simulink model "SelectiveHarmonicsEliminationfor1phbridgeinverter"  (R2023a)
settings: Solver=VariableStepAuto  StartTime=0.0  StopTime=0.2  RelTol=1e-3
values from neighbouring files (symbols this model uses):
  alpha = [alpha1;alpha2;alpha3;alpha4;alpha5]*180/pi    [SHEnewtonraphson.m]
libraries: spsIGBTDiodeLib x4, simulink x2, spsDCVoltageSourceLib x1, spsGroundLib x1, spsSeriesRLCBranchLib x1, spsVoltageMeasurementLib x1, sps_lib x1
settings Model: Creator=User  LastModifiedBy=User

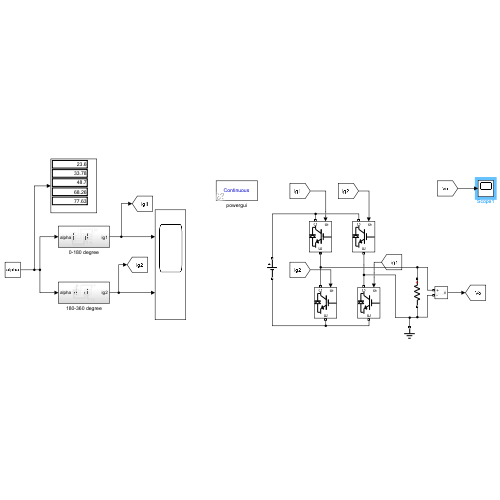
[thumbnail: Simulink's stored preview of the top-level diagram]
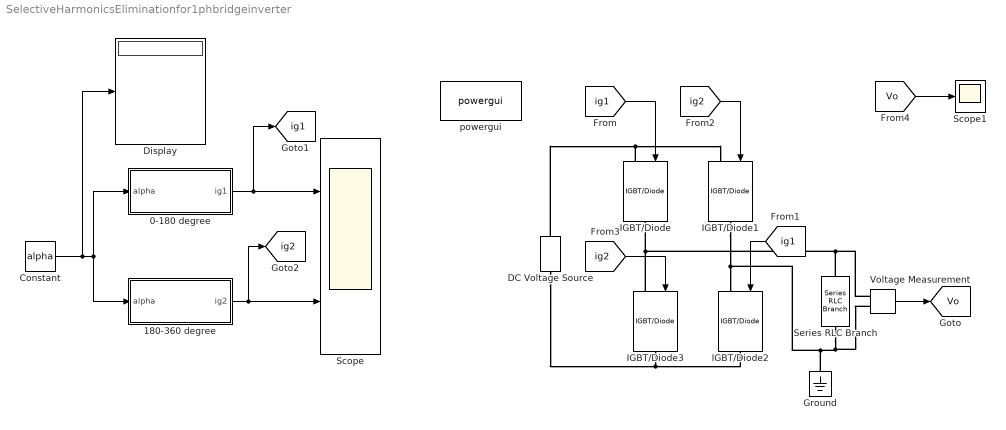
== system SelectiveHarmonicsEliminationfor1phbridgeinverter ==
  0-180 degree : Subsystem
  180-360 degree : Subsystem
  Constant : Constant  Value=alpha
  DC Voltage Source : spsDCVoltageSourceLib/DC Voltage Source  Amplitude=200  Measurements=None
  Display : Display
  Ground : spsGroundLib/Ground  LConnTagsString=a
  IGBT/Diode{,1..3} (4 alike) : spsIGBTDiodeLib/IGBT//Diode  Ron=1e-3  Rs=1e5  Cs=inf  Measurements=off
  Scope : Scope  NumInputPorts=2
  Scope1 : Scope
  Series RLC Branch : spsSeriesRLCBranchLib/Series RLC Branch  LConnTagsString=__new0  RConnTagsString=__new0  BranchType=R  Resistance=10  Inductance=1e-3  SetiL0=off  InitialCurrent=0  Capacitance=1e-6  Setx0=off  InitialVoltage=0  Measurements=None
  Voltage Measurement : spsVoltageMeasurementLib/Voltage Measurement  PhasorSimulation=off  OutputType=Complex  PSBequivalent=0
  powergui : sps_lib/powergui  Priority=1  SimulationMode=Continuous  SampleTime=50e-6  frequency=60  Iterations=50  frequencyindice=0  Pbase=100e6  ErrMax=1e-4  UnitsV=kV  UnitsW=MW  buscounter=0  FunctionMessages=off  echomessages=off  EnableUseOfTLC=off  CurrentSourceSwitches=off  DisableSnubberDevices=off  DisableRonSwitches=off  DisableVfSwitches=off  DisplayEquations=off  AutomaticDiscreteSolvers=off  SolverType=Tustin/Backward Euler (TBE)  Interpol=off  ExternalGateDelay=off  methode=off  Ts=100  x0status=blocks  SPID=on  SwTol=0  HookPort=off  NonlinearTolerance=1e-4  nMaxIteration=100  ContinueOnMaxIteration=off  RestoreLinks=warning  ResistiveCurrentMeasurement=off  Frange=[0:2:500]  Ylog=off  Xlog=on  ShowGrid=off  save=off  variable=ZData  structure=0  ZoomFFT=off  StartTime=0.0  cycles=1  DisplayStyle=1  fundamental=60  FreqAxis=off  MaxFrequency=1000  frequencyindicesteady=1  RmsSteady=1  display=off
  tag scope: Vo=global, ig1=global, ig2=global
  wires:
  Voltage Measurement/1 -> [Vo]
  Constant/1 -> Display/1, 180-360 degree/1(alpha), 0-180 degree/1(alpha)
  180-360 degree/1(ig2) -> Scope/2, [ig2]
  0-180 degree/1(ig1) -> [ig1], Scope/1
  [ig1] -> IGBT/Diode/1
  [ig1] -> IGBT/Diode2/1
  [ig2] -> IGBT/Diode1/1
  [ig2] -> IGBT/Diode3/1
  [Vo] -> Scope1/1
  connections:
  IGBT/Diode1/RConn1 -- Ground/LConn1 -- Voltage Measurement/LConn2 -- Series RLC Branch/RConn1 -- IGBT/Diode2/LConn1
  IGBT/Diode3/LConn1 -- Series RLC Branch/LConn1 -- Voltage Measurement/LConn1 -- IGBT/Diode/RConn1
  IGBT/Diode/LConn1 -- IGBT/Diode1/LConn1 -- DC Voltage Source/RConn1
  IGBT/Diode3/RConn1 -- IGBT/Diode2/RConn1 -- DC Voltage Source/LConn1

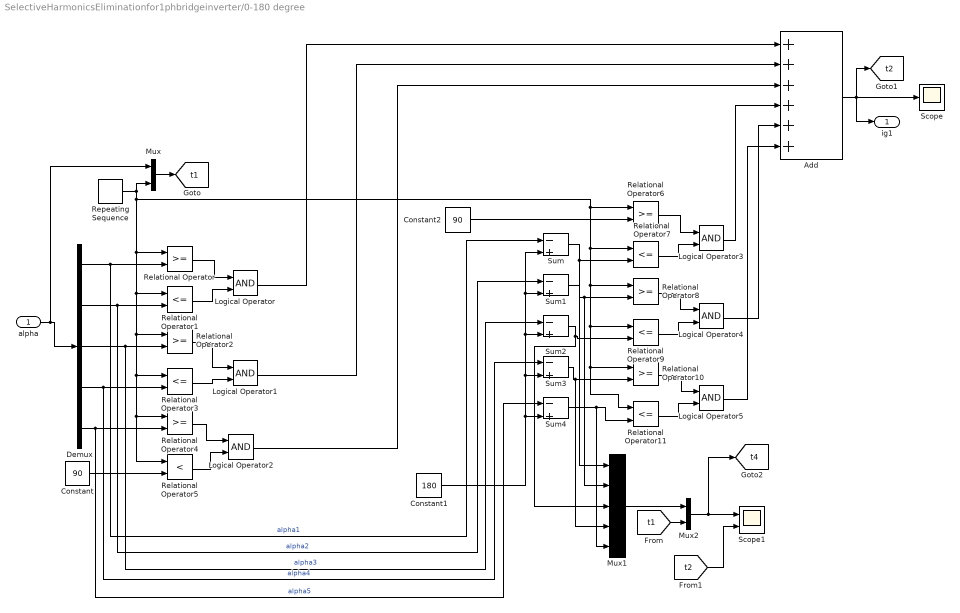
== system SelectiveHarmonicsEliminationfor1phbridgeinverter/0-180 degree ==
  alpha : Inport
  Add : Sum  Inputs=++++++  OutDataTypeStr=Inherit: Inherit via back propagation
  Constant : Constant  Value=90
  Constant1 : Constant  Value=180
  Constant2 : Constant  Value=90
  Demux : Demux  Outputs=5
  Logical Operator{,1..5} (6 alike) : Logic  AllPortsSameDT=off  OutDataTypeStr=boolean
  Mux : Mux  Inputs=2
  Mux1 : Mux  Inputs=5
  Mux2 : Mux  Inputs=2
  Relational Operator{,2,4,6,8,10} (6 alike) : RelationalOperator  OutDataTypeStr=boolean  RndMeth=Simplest  InputSameDT=off
  Relational Operator{1,3,7,9,11} (5 alike) : RelationalOperator  Operator=<=  OutDataTypeStr=boolean  RndMeth=Simplest  InputSameDT=off
  Relational Operator5 : RelationalOperator  Operator=<  OutDataTypeStr=boolean  RndMeth=Simplest  InputSameDT=off
  Repeating Sequence : simulink/Sources/Repeating Sequence  rep_seq_t=[0 1]*0.02  rep_seq_y=[0 360]
  Scope : Scope
  Scope1 : Scope  NumInputPorts=2
  Sum{,1..4} (5 alike) : Sum  Inputs=|-+
  ig1 : Outport
  tag scope: t1=global, t2=global, t4=global
  wires:
  alpha/1 -> Mux/1, Demux/1
  Relational Operator/1 -> Logical Operator/1
  Relational Operator1/1 -> Logical Operator/2
  Relational Operator2/1 -> Logical Operator1/1
  Relational Operator3/1 -> Logical Operator1/2
  Relational Operator4/1 -> Logical Operator2/1
  Relational Operator5/1 -> Logical Operator2/2
  Demux/1 -> Relational Operator/2, Sum/1  "alpha1"
  Demux/2 -> Sum1/1, Relational Operator1/2  "alpha2"
  Demux/3 -> Sum2/1, Relational Operator2/2  "alpha3"
  Demux/4 -> Sum3/1, Relational Operator3/2  "alpha4"
  Demux/5 -> Sum4/1, Relational Operator4/2  "alpha5"
  Constant/1 -> Relational Operator5/2
  Mux/1 -> [t1]
  Repeating Sequence/1 -> Mux/2, Relational Operator5/1, Relational Operator4/1, Relational Operator3/1, Relational Operator2/1, Relational Operator1/1, Relational Operator/1, Relational Operator10/1, Relational Operator11/1, Relational Operator9/1, Relational Operator8/1, Relational Operator7/1, Relational Operator6/1
  Constant1/1 -> Sum/2, Sum1/2, Sum2/2, Sum3/2, Sum4/2
  Relational Operator6/1 -> Logical Operator3/1
  Relational Operator7/1 -> Logical Operator3/2
  Relational Operator8/1 -> Logical Operator4/1
  Relational Operator9/1 -> Logical Operator4/2
  Relational Operator10/1 -> Logical Operator5/1
  Relational Operator11/1 -> Logical Operator5/2
  Sum/1 -> Mux1/1, Relational Operator7/2
  Constant2/1 -> Relational Operator6/2
  Sum1/1 -> Mux1/2, Relational Operator8/2
  Sum2/1 -> Mux1/3, Relational Operator9/2
  Sum3/1 -> Mux1/4, Relational Operator10/2
  Sum4/1 -> Mux1/5, Relational Operator11/2
  Logical Operator/1 -> Add/1
  Logical Operator1/1 -> Add/2
  Logical Operator2/1 -> Add/3
  Logical Operator3/1 -> Add/4
  Logical Operator4/1 -> Add/5
  Logical Operator5/1 -> Add/6
  Add/1 -> ig1/1, Scope/1, [t2]
  Mux1/1 -> Mux2/1
  [t1] -> Mux2/2
  Mux2/1 -> [t4], Scope1/1
  [t2] -> Scope1/2

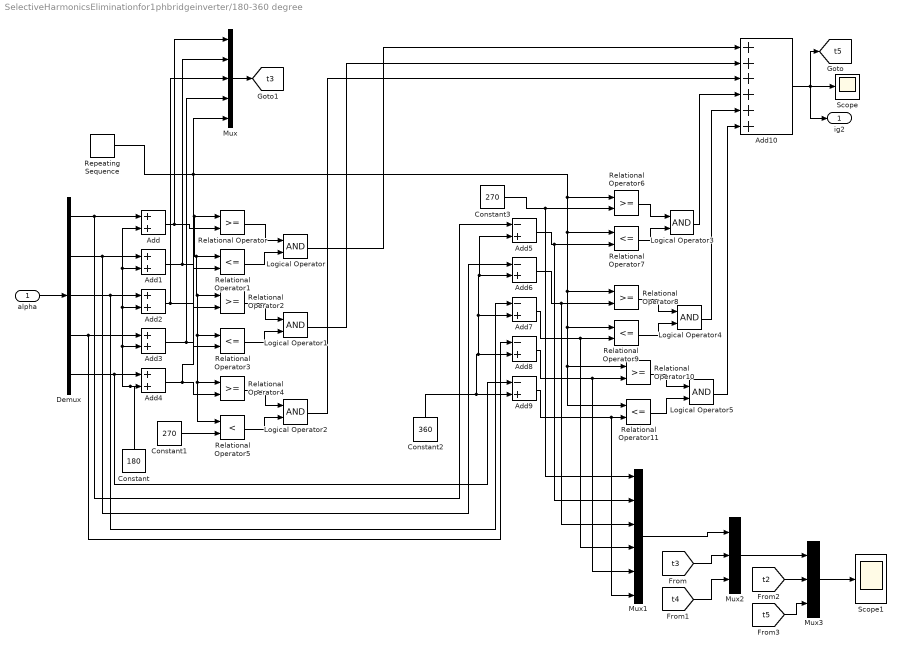
== system SelectiveHarmonicsEliminationfor1phbridgeinverter/180-360 degree ==
  alpha : Inport
  Add{,1..4} (5 alike) : Sum
  Add10 : Sum  Inputs=++++++  OutDataTypeStr=Inherit: Inherit via back propagation
  Add{5..9} (5 alike) : Sum  Inputs=-+
  Constant : Constant  Value=180
  Constant1 : Constant  Value=270
  Constant2 : Constant  Value=360
  Constant3 : Constant  Value=270
  Demux : Demux  Outputs=5
  Logical Operator{,1..5} (6 alike) : Logic  AllPortsSameDT=off  OutDataTypeStr=boolean
  Mux : Mux  Inputs=5
  Mux1 : Mux  Inputs=6
  Mux2 : Mux  Inputs=3
  Mux3 : Mux  Inputs=3
  Relational Operator{,2,4,6,8,10} (6 alike) : RelationalOperator  OutDataTypeStr=boolean  RndMeth=Simplest  InputSameDT=off
  Relational Operator{1,3,7,9,11} (5 alike) : RelationalOperator  Operator=<=  OutDataTypeStr=boolean  RndMeth=Simplest  InputSameDT=off
  Relational Operator5 : RelationalOperator  Operator=<  OutDataTypeStr=boolean  RndMeth=Simplest  InputSameDT=off
  Repeating Sequence : simulink/Sources/Repeating Sequence  rep_seq_t=[0 1]*0.02  rep_seq_y=[0 360]
  Scope : Scope
  Scope1 : Scope
  ig2 : Outport
  tag scope: t3=global, t5=global
  wires:
  alpha/1 -> Demux/1
  Demux/2 -> Add6/1, Add1/1
  Demux/1 -> Add5/1, Add/1
  Demux/3 -> Add7/1, Add2/1
  Demux/4 -> Add8/1, Add3/1
  Demux/5 -> Add9/1, Add4/1
  Constant/1 -> Add3/2, Add2/2, Add1/2, Add/2, Add4/2
  Relational Operator/1 -> Logical Operator/1
  Relational Operator1/1 -> Logical Operator/2
  Relational Operator2/1 -> Logical Operator1/1
  Relational Operator3/1 -> Logical Operator1/2
  Relational Operator4/1 -> Logical Operator2/1
  Relational Operator5/1 -> Logical Operator2/2
  Add/1 -> Mux/1, Relational Operator/2
  Add2/1 -> Relational Operator2/2, Mux/3
  Add3/1 -> Relational Operator3/2, Mux/4
  Add4/1 -> Mux/5, Relational Operator4/2
  Repeating Sequence/1 -> Relational Operator5/1, Relational Operator4/1, Relational Operator3/1, Relational Operator2/1, Relational Operator1/1, Relational Operator/1, Relational Operator10/1, Relational Operator11/1, Relational Operator9/1, Relational Operator8/1, Relational Operator7/1, Relational Operator6/1
  Constant1/1 -> Relational Operator5/2
  Constant2/1 -> Add5/2, Add6/2, Add7/2, Add8/2, Add9/2
  Relational Operator6/1 -> Logical Operator3/1
  Relational Operator7/1 -> Logical Operator3/2
  Relational Operator9/1 -> Logical Operator4/2
  Relational Operator8/1 -> Logical Operator4/1
  Relational Operator11/1 -> Logical Operator5/2
  Relational Operator10/1 -> Logical Operator5/1
  Add5/1 -> Mux1/2, Relational Operator7/2
  Add6/1 -> Mux1/3, Relational Operator8/2
  Add8/1 -> Mux1/5, Relational Operator10/2
  Add9/1 -> Mux1/6, Relational Operator11/2
  Constant3/1 -> Mux1/1, Relational Operator6/2
  Logical Operator3/1 -> Add10/4
  Logical Operator4/1 -> Add10/5
  Logical Operator5/1 -> Add10/6
  Logical Operator/1 -> Add10/1
  Logical Operator1/1 -> Add10/2
  Logical Operator2/1 -> Add10/3
  Add10/1 -> [t5], Scope/1, ig2/1
  Add1/1 -> Mux/2, Relational Operator1/2
  Mux/1 -> [t3]
  Add7/1 -> Mux1/4, Relational Operator9/2
  Mux1/1 -> Mux2/1
  [t3] -> Mux2/2
  Mux2/1 -> Mux3/1
  [t4] -> Mux2/3
  [t2] -> Mux3/2
  [t5] -> Mux3/3
  Mux3/1 -> Scope1/1
